simulink model "HILModel_flightgear"  (Simulink 7.8)
settings: Solver=ode4  StartTime=0.0  StopTime=inf  FixedStep=SampleT  RelTol=1e-3
InitFcn:
  | clc
  | hilInit
  | launchFlightgear
values from neighbouring files (symbols this model uses):
  Euler_0 = [0; 0*pi/180; 0*pi/180]'    [hilInit.m]
  HIL_K = 3    [hilInit.m]
  Pos_0 = [0; 0; 150]'    [hilInit.m]
  SampleT = 0.005    [hilInit.m]
  Vb_0 = [ 17; 0; 0]'    [hilInit.m]
  windBase = 3.5    [hilInit.m]
undefined symbols (not defined in the file or in its folder): A1, Apolar, barAdjust, baroOffset, baroScale, barTGain2, barTMean2, bPWMda, bPWMde, bPWMdr, bPWMdt, CD0, chord, CL0, CLa, CLa_dot, Clb, ClDa, CLDe, CLDf, ClDr, clock, Clp, CLq, Clr, Cm0, Cma, CmDe, CmDf, Cmq, Cnb, CnDa, CnDr, Cnp, Cnr, cubeAccelGain16405, cubeGyroGain16405, cubeMagGain16405, CYb, CYDr, da_failamp, da_failbias, da_failper, daL_fail, daR_fail, DiscIntNeverNeededParam, dr_fail, Earth, elarm, F, GS_location, ISA_g, Ixx, Iyy, Izz, Light, mass, MIL, MinThK, mPWMda ... (+14)
libraries: simulink x30, aerolibconvert2 x11, xpclib x8, aerolibactuator x5, aerolibwind2 x2, dspmtrx3 x2, aerolibfltsims x2, aerolibtransform2 x1, aerolibobsolete x1, aerolibatmos2 x1, aerolibanimutils x1
(part 3 of 3)

== system HILModel_flightgear/6DOF Model/Plant/Forces and Moments/Body Frame F & M/Wind frame F& M/Lateral Channel/Cn/yaw factors ==
  p,q,r : Inport
  Airspeed : Inport  Port=2
  Cnp1 : simulink/Math Operations/Slider Gain  low=-500  gain=1  high=50
  Cnr1 : simulink/Math Operations/Slider Gain  low=0  gain=1  high=500
  Constant : Constant  Value=Cnp
  Constant1 : Constant  Value=Cnr
  Get p : Selector  InputPortWidth=3  IndexOptions=Index vector (dialog)  Indices=1  OutputSizes=[(-2)]
  Get r : Selector  InputPortWidth=3  IndexOptions=Index vector (dialog)  Indices=3  OutputSizes=[(-2)]
  Product : Product  SaturateOnIntegerOverflow=on  OutDataTypeStr=Inherit: Same as first input
  Product1 : Product  SaturateOnIntegerOverflow=on  OutDataTypeStr=Inherit: Same as first input
  roll rate fact : Subsystem
  yaw rate fact : Subsystem
  Cnp : Outport
  Cnr : Outport  Port=2
  wires:
  Product/1 -> Cnp/1
  Product1/1 -> Cnr/1
  Constant1/1 -> Cnr1/1
  Cnr1/1 -> Product1/1
  yaw rate fact/1(Yaw Rate Fac) -> Product1/2
  Constant/1 -> Cnp1/1
  Cnp1/1 -> Product/1
  roll rate fact/1(Roll Rate Fac) -> Product/2
  Get p/1 -> roll rate fact/1(p)
  p,q,r/1 -> Get p/1, Get r/1
  Get r/1 -> yaw rate fact/1(r)
  Airspeed/1 -> roll rate fact/2(Airspeed), yaw rate fact/2(Airspeed)

== system HILModel_flightgear/6DOF Model/Plant/Forces and Moments/Body Frame F & M/Wind frame F& M/Longitudinal Channel/CL/Lift due to pitch rate ==
  p,q,r : Inport
  Airspeed : Inport  Port=2
  Constant : Constant  Value=CLq
  Get q : Selector  InputPortWidth=3  IndexOptions=Index vector (dialog)  Indices=2  OutputSizes=[(-2)]
  Product : Product  SaturateOnIntegerOverflow=on  OutDataTypeStr=Inherit: Same as first input
  pitch rate factor : Subsystem
  tune CLq : simulink/Math Operations/Slider Gain  low=0  gain=1  high=2000
  CLq : Outport
  wires:
  tune CLq/1 -> Product/1
  pitch rate factor/1(Pitch Rate Fac) -> Product/2
  Constant/1 -> tune CLq/1
  Product/1 -> CLq/1
  p,q,r/1 -> Get q/1
  Get q/1 -> pitch rate factor/1(q)
  Airspeed/1 -> pitch rate factor/2(Airspeed)

== system HILModel_flightgear/6DOF Model/Plant/Forces and Moments/Body Frame F & M/Wind frame F& M/Lateral Channel/Cl/roll factors/roll rate fact ==
  p : Inport
  Airspeed : Inport  Port=2
  Cmq1 : Constant  Value=.5
  Cmq2 : Constant  Value=span
  Product : Product  Inputs=***/  SaturateOnIntegerOverflow=on  OutDataTypeStr=Inherit: Same as first input
  Roll Rate Fac : Outport
  wires:
  Product/1 -> Roll Rate Fac/1
  p/1 -> Product/1
  Cmq1/1 -> Product/2
  Cmq2/1 -> Product/3
  Airspeed/1 -> Product/4

== system HILModel_flightgear/6DOF Model/Plant/Forces and Moments/Body Frame F & M/Wind frame F& M/Lateral Channel/Cl/roll factors/yaw rate fact ==
  r : Inport
  Airspeed : Inport  Port=2
  Cmq1 : Constant  Value=.5
  Cmq2 : Constant  Value=span
  Product : Product  Inputs=***/  SaturateOnIntegerOverflow=on  OutDataTypeStr=Inherit: Same as first input
  Yaw Rate Fac : Outport
  wires:
  r/1 -> Product/1
  Cmq1/1 -> Product/2
  Airspeed/1 -> Product/4
  Cmq2/1 -> Product/3
  Product/1 -> Yaw Rate Fac/1

== system HILModel_flightgear/6DOF Model/Plant/Forces and Moments/Body Frame F & M/Wind frame F& M/Lateral Channel/Cn/yaw factors/roll rate fact ==
  p : Inport
  Airspeed : Inport  Port=2
  Cmq1 : Constant  Value=.5
  Cmq2 : Constant  Value=span
  Product : Product  Inputs=***/  SaturateOnIntegerOverflow=on  OutDataTypeStr=Inherit: Same as first input
  Roll Rate Fac : Outport
  wires:
  Product/1 -> Roll Rate Fac/1
  p/1 -> Product/1
  Cmq1/1 -> Product/2
  Cmq2/1 -> Product/3
  Airspeed/1 -> Product/4

== system HILModel_flightgear/6DOF Model/Plant/Forces and Moments/Body Frame F & M/Wind frame F& M/Lateral Channel/Cn/yaw factors/yaw rate fact ==
  r : Inport
  Airspeed : Inport  Port=2
  Cmq3 : Constant  Value=.5
  Cmq4 : Constant  Value=span
  Product1 : Product  Inputs=***/  SaturateOnIntegerOverflow=on  OutDataTypeStr=Inherit: Same as first input
  Yaw Rate Fac : Outport
  wires:
  Product1/1 -> Yaw Rate Fac/1
  r/1 -> Product1/1
  Cmq3/1 -> Product1/2
  Cmq4/1 -> Product1/3
  Airspeed/1 -> Product1/4

== system HILModel_flightgear/6DOF Model/Plant/Forces and Moments/Body Frame F & M/Wind frame F& M/Longitudinal Channel/CL/Lift due to pitch rate/pitch rate factor ==
  q : Inport
  Airspeed : Inport  Port=2
  Cmq2 : Constant  Value=chord
  Product : Product  Inputs=**/  SaturateOnIntegerOverflow=on  OutDataTypeStr=Inherit: Same as first input
  Pitch Rate Fac : Outport
  wires:
  Product/1 -> Pitch Rate Fac/1
  q/1 -> Product/1
  Airspeed/1 -> Product/3
  Cmq2/1 -> Product/2

== matlab function 6DOF Model/Plant/Get GPS/Embedded MATLAB Function1 ==
  data: cog output double; Vn input double; Ve input double
function cog = getCOG(Vn, Ve)
% This block supports an embeddable subset of the MATLAB language.
% See the help menu for details. 

cog = atan2(Ve,Vn);
if cog < 0;
    cog = cog + 2*pi;
end
